simulink model "ejemplo_simulink_completo_vel_lineal"  (R2018a)
settings: Solver=FixedStepDiscrete  StartTime=0.0  StopTime=inf  FixedStep=0.001  RelTol=1e-3  EnableMultiTasking=on
libraries: aerolibanimutils x1
settings Model: Creator=PC  LastModifiedBy=emder
settings OptimizationCC: LifeSpan=inf
settings DebuggingCC: SFUnexpectedBacktrackingDiag=warning  SFNoUnconditionalDefaultTransitionDiag=warning  SFExecutionAtInitializationDiag=none
settings CodeAppCC: StateflowObjectComments=on
settings GRTTargetCC: TargetLangStandard=C89/C90 (ANSI)  GeneratePreprocessorConditionals=Disable all
settings ConfigComp: CovMetricSettings=dw  CovHtmlReporting=on  CovSaveCumulativeToWorkspaceVar=on  CovSaveSingleToWorkspaceVar=on  CovExternalEMLEnable=off

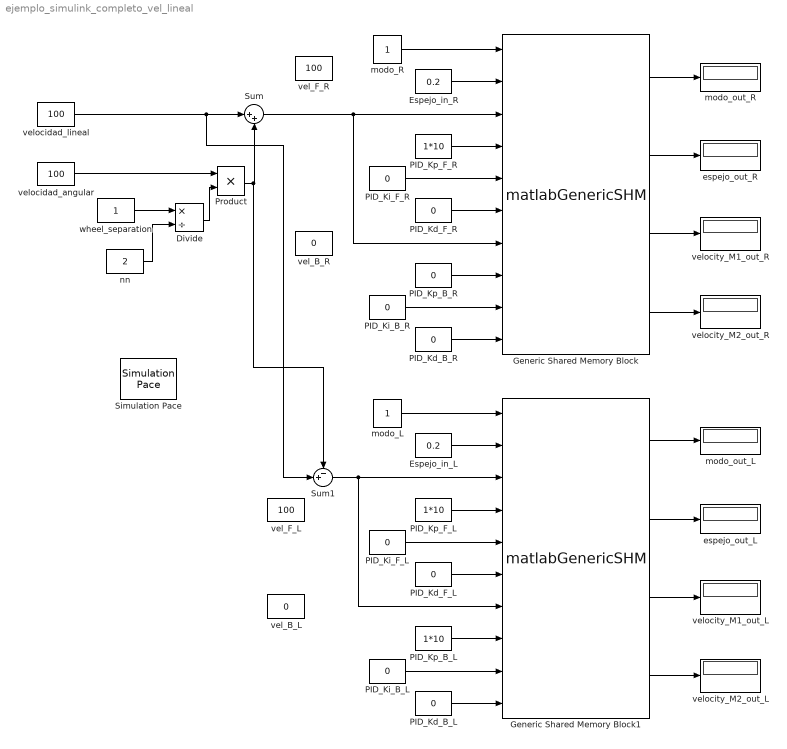
== system ejemplo_simulink_completo_vel_lineal ==
  Divide : Product  Inputs=*/
  Espejo_in_L : Constant  Value=0.2  OutDataTypeStr=single
  Espejo_in_R : Constant  Value=0.2  OutDataTypeStr=single
  Generic Shared Memory Block : S-Function  FunctionName=matlabGenericSHM  Parameters=nombre,dispositivo,vecE,vecS,tipoE,tipoS,ts  SFunctionDeploymentMode=off  EnableBusSupport=off  mask(Generic Share Memory block V2.0){nombre='ARDUINO', dispositivo=1, vecE=[1 1 1 1 1 1 1 1 1 1], vecS=[1 1 1 1], tipoE=['f' 'f' 'f' 'f' 'f' 'f' 'f' 'f' 'f' 'f'], tipoS=['f' 'f' 'f' 'f'], ts=-1}
      mask prompts: nombre "Share Memory base name"; dispositivo "Device Number"; vecE "Sizes input vector"; vecS "Sizes output vector"; tipoE "Data Types Inputs"; tipoS "Data Types Outputs"; ts "Sample Time"
      mask help:
      | This block allows Simulink communication with external processes through shared memory. It works on Unix and Windows.
      | More information in Help.
      mask Help:
      | Share Memory base name (nombre): It's the base string of share memory ej 'robot'
      | Device Number (dispositivo): integer that identifies the device between multiple in use
      | Two shared memorys are created with names:
      | "%name_entrada_%dispositivo" for the device input (writing)
      | "%name_salida_%dispositivo" for the device output (reading)
      | Sizes input vector (vecE)  : array that specify the number of inputs (array dimension) and the inputs size (array values)
      | Sizes output vector  (vecS): array that specify the number of outputs (array dimension) and the outputs size (array values)
      | Data types input(tipoE): char array that specify each input types
      | Data types output (tipoS): char array that specify each output types
      | Allowed types are:
      | ('f'=float, 'd'=double, 'i'=int32, 'c'=char, 'C'= unsigned char, 'I'=unsigned int)
      | Example.
      | Suppose the following parameters:
      | nombre='exampleMemory'
      | dispositivo=10
      | vecE=[3 2 1]
      | vecS=[6 5 7 8]
      | tipoE=['f' 'I' 'c']
      | tipoS=['C' 'i' 'd' 'd']
      | 
      | Two Share Memories are created with names:
      | "exampleMemory_entrada_10" (block input)
      | "exampleMemory_salida_10"  (block output)
      | 3 inputs are created:
      |  1° Dimension 3, type "unsigned char"
      |  2° Dimension 2, type "int"
      |  3° Dimension 1, type "char"
      | 4 outputs are created:
      |  1° Dimension 6, type "float"
      |  2° Dimension 5, type "unsigned int"
      |  3° Dimension 7, type "double"
      |  3° Dimension 8, type "double"
      mask Display: image('shmem.jpg')
  Generic Shared Memory Block1 : S-Function  FunctionName=matlabGenericSHM  Parameters=nombre,dispositivo,vecE,vecS,tipoE,tipoS,ts  SFunctionDeploymentMode=off  EnableBusSupport=off  mask(Generic Share Memory block V2.0){nombre='ARDUINO', dispositivo=2, vecE=[1 1 1 1 1 1 1 1 1 1], vecS=[1 1 1 1], tipoE=['f' 'f' 'f' 'f' 'f' 'f' 'f' 'f' 'f' 'f'], tipoS=['f' 'f' 'f' 'f'], ts=-1}
      mask prompts: nombre "Share Memory base name"; dispositivo "Device Number"; vecE "Sizes input vector"; vecS "Sizes output vector"; tipoE "Data Types Inputs"; tipoS "Data Types Outputs"; ts "Sample Time"
      mask help:
      | This block allows Simulink communication with external processes through shared memory. It works on Unix and Windows.
      | More information in Help.
      mask Help:
      | Share Memory base name (nombre): It's the base string of share memory ej 'robot'
      | Device Number (dispositivo): integer that identifies the device between multiple in use
      | Two shared memorys are created with names:
      | "%name_entrada_%dispositivo" for the device input (writing)
      | "%name_salida_%dispositivo" for the device output (reading)
      | Sizes input vector (vecE)  : array that specify the number of inputs (array dimension) and the inputs size (array values)
      | Sizes output vector  (vecS): array that specify the number of outputs (array dimension) and the outputs size (array values)
      | Data types input(tipoE): char array that specify each input types
      | Data types output (tipoS): char array that specify each output types
      | Allowed types are:
      | ('f'=float, 'd'=double, 'i'=int32, 'c'=char, 'C'= unsigned char, 'I'=unsigned int)
      | Example.
      | Suppose the following parameters:
      | nombre='exampleMemory'
      | dispositivo=10
      | vecE=[3 2 1]
      | vecS=[6 5 7 8]
      | tipoE=['f' 'I' 'c']
      | tipoS=['C' 'i' 'd' 'd']
      | 
      | Two Share Memories are created with names:
      | "exampleMemory_entrada_10" (block input)
      | "exampleMemory_salida_10"  (block output)
      | 3 inputs are created:
      |  1° Dimension 3, type "unsigned char"
      |  2° Dimension 2, type "int"
      |  3° Dimension 1, type "char"
      | 4 outputs are created:
      |  1° Dimension 6, type "float"
      |  2° Dimension 5, type "unsigned int"
      |  3° Dimension 7, type "double"
      |  3° Dimension 8, type "double"
      mask Display: image('shmem.jpg')
  PID_Kd_B_L : Constant  Value=0  OutDataTypeStr=single
  PID_Kd_B_R : Constant  Value=0  OutDataTypeStr=single
  PID_Kd_F_L : Constant  Value=0  OutDataTypeStr=single
  PID_Kd_F_R : Constant  Value=0  OutDataTypeStr=single
  PID_Ki_B_L : Constant  Value=0  OutDataTypeStr=single
  PID_Ki_B_R : Constant  Value=0  OutDataTypeStr=single
  PID_Ki_F_L : Constant  Value=0  OutDataTypeStr=single
  PID_Ki_F_R : Constant  Value=0  OutDataTypeStr=single
  PID_Kp_B_L : Constant  Value=1*10  OutDataTypeStr=single
  PID_Kp_B_R : Constant  Value=0  OutDataTypeStr=single
  PID_Kp_F_L : Constant  Value=1*10  OutDataTypeStr=single
  PID_Kp_F_R : Constant  Value=1*10  OutDataTypeStr=single
  Product : Product
  Simulation Pace : aerolibanimutils/Simulation Pace  SimulationPace=1  SleepMode=MATLAB Thread  OutputPaceError=off  SampleTime=-1
  Sum : Sum  Inputs=|++
  Sum1 : Sum  Inputs=-+|
  espejo_out_L : Display
  espejo_out_R : Display
  modo_L : Constant  OutDataTypeStr=single  SampleTime=-1
  modo_R : Constant  OutDataTypeStr=single  SampleTime=-1
  modo_out_L : Display
  modo_out_R : Display
  nn : Constant  Value=2  OutDataTypeStr=single
  vel_B_L : Constant  Value=0  OutDataTypeStr=single
  vel_B_R : Constant  Value=0  OutDataTypeStr=single
  vel_F_L : Constant  Value=100  OutDataTypeStr=single
  vel_F_R : Constant  Value=100  OutDataTypeStr=single
  velocidad_angular : Constant  Value=100  OutDataTypeStr=single
  velocidad_lineal : Constant  Value=100  OutDataTypeStr=single
  velocity_M1_out_L : Display
      settings: Decimation=3
  "velocity_M1_out_R " : Display
      settings: Decimation=3
  velocity_M2_out_L : Display
  velocity_M2_out_R : Display
  wheel_separation : Constant  OutDataTypeStr=single
  wires:
  modo_R/1 -> Generic Shared Memory Block/1
  Generic Shared Memory Block/1 -> modo_out_R/1
  Generic Shared Memory Block/2 -> espejo_out_R/1
  Espejo_in_R/1 -> Generic Shared Memory Block/2
  Generic Shared Memory Block/3 -> "velocity_M1_out_R "/1
  Generic Shared Memory Block/4 -> velocity_M2_out_R/1
  velocidad_angular/1 -> Product/1
  Divide/1 -> Product/2
  wheel_separation/1 -> Divide/1
  nn/1 -> Divide/2
  velocidad_lineal/1 -> Sum1/2, Sum/1
  Product/1 -> Sum1/1, Sum/2
  Sum/1 -> Generic Shared Memory Block/3, Generic Shared Memory Block/7
  PID_Kp_F_R/1 -> Generic Shared Memory Block/4
  PID_Ki_F_R/1 -> Generic Shared Memory Block/5
  PID_Kd_F_R/1 -> Generic Shared Memory Block/6
  PID_Kp_B_R/1 -> Generic Shared Memory Block/8
  PID_Ki_B_R/1 -> Generic Shared Memory Block/9
  PID_Kd_B_R/1 -> Generic Shared Memory Block/10
  PID_Ki_B_L/1 -> Generic Shared Memory Block1/9
  Generic Shared Memory Block1/2 -> espejo_out_L/1
  PID_Kd_B_L/1 -> Generic Shared Memory Block1/10
  Espejo_in_L/1 -> Generic Shared Memory Block1/2
  Generic Shared Memory Block1/4 -> velocity_M2_out_L/1
  Generic Shared Memory Block1/3 -> velocity_M1_out_L/1
  Generic Shared Memory Block1/1 -> modo_out_L/1
  modo_L/1 -> Generic Shared Memory Block1/1
  PID_Kp_F_L/1 -> Generic Shared Memory Block1/4
  PID_Kp_B_L/1 -> Generic Shared Memory Block1/8
  PID_Kd_F_L/1 -> Generic Shared Memory Block1/6
  Sum1/1 -> Generic Shared Memory Block1/3, Generic Shared Memory Block1/7
  PID_Ki_F_L/1 -> Generic Shared Memory Block1/5
